simulink model "01_zvzvsspd"  (R2025a)
settings: Solver=FixedStepDiscrete  StartTime=0.0  StopTime=10  FixedStep=Ts  RelTol=1e-3
model workspace (MATLAB code in the model file):
  | N = 31;
  | n = 0:N-1;
  | sigma = (N-1)/6;
  | g = exp(-0.5*((n-(N-1)/2)/sigma).^2);
  | h = g / sum(g);
undefined symbols (not defined in the file): DiscIntNeverNeededParam, Ts
settings Model: Creator=wattanakhonvipanna  LastModifiedBy=wattanakhonvipanna

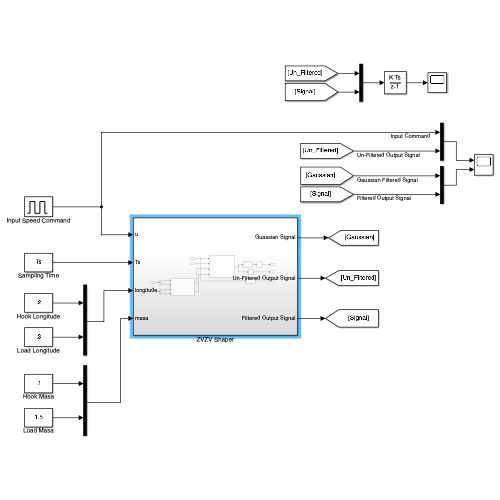
[thumbnail: Simulink's stored preview of the top-level diagram]
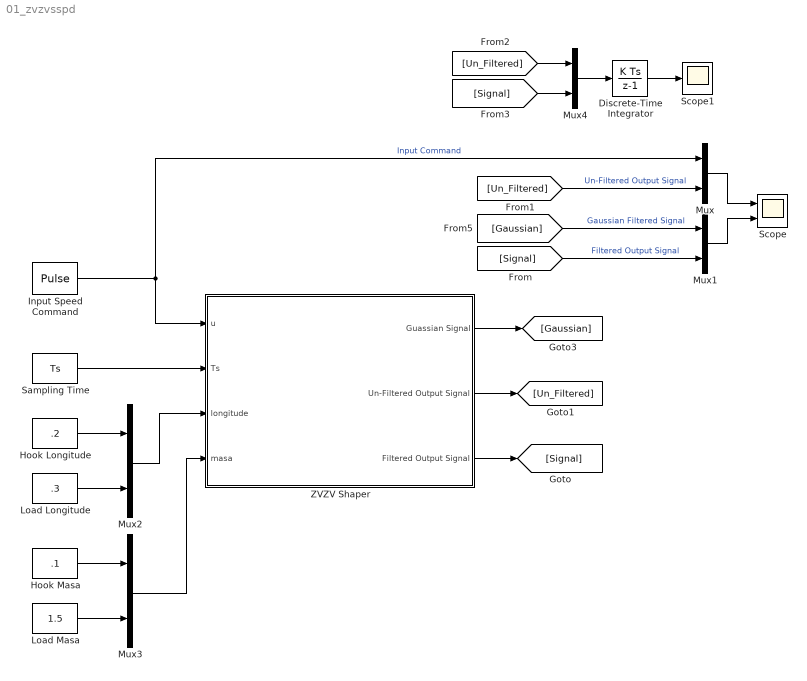
== system 01_zvzvsspd ==
  Discrete-Time Integrator : DiscreteIntegrator  SampleTime=-1  ICPrevOutput=DiscIntNeverNeededParam  ICPrevScaledInput=DiscIntNeverNeededParam
  Hook Longitude : Constant  Value=.2
  Hook Masa : Constant  Value=.1
  Input Speed Command : DiscretePulseGenerator  PulseType=Time based  Amplitude=0.2  Period=10  PulseWidth=50
  Load Longitude : Constant  Value=.3
  Load Masa : Constant  Value=1.5
  Mux{,1..4} (5 alike) : Mux  Inputs=2
  Sampling Time : Constant  Value=Ts
  Scope : Scope  NumInputPorts=2
      settings: ActiveDisplayYMinimum=-0.024999999999999998  ActiveDisplayYMaximum=0.22500000000000003  YLabel=speed (ms^-^1)
  Scope1 : Scope
      settings: ActiveDisplayYMinimum=-0.31249999999999656  ActiveDisplayYMaximum=2.8124999999999694  YLabel=position (m)  DataLoggingVariableName=ScopeData2
  ZVZV Shaper : Subsystem
  wires:
  Sampling Time/1 -> ZVZV Shaper/2(Ts)
  ZVZV Shaper/3(Filtered Output Signal) -> [Signal]
  ZVZV Shaper/2(Un-Filtered Output Signal) -> [Un_Filtered]
  [Un_Filtered] -> Mux/2  "Un-Filtered Output Signal"
  Mux/1 -> Scope/1
  Input Speed Command/1 -> ZVZV Shaper/1(u), Mux/1  "Input Command"
  Mux1/1 -> Scope/2
  [Gaussian] -> Mux1/1  "Gaussian Filtered Signal"
  [Signal] -> Mux1/2  "Filtered Output Signal"
  ZVZV Shaper/1(Guassian Signal) -> [Gaussian]
  Mux2/1 -> ZVZV Shaper/3(longitude)
  Hook Longitude/1 -> Mux2/1
  Load Longitude/1 -> Mux2/2
  Load Masa/1 -> Mux3/2
  Hook Masa/1 -> Mux3/1
  Mux3/1 -> ZVZV Shaper/4(masa)
  Mux4/1 -> Discrete-Time Integrator/1
  [Un_Filtered] -> Mux4/1
  [Signal] -> Mux4/2
  Discrete-Time Integrator/1 -> Scope1/1

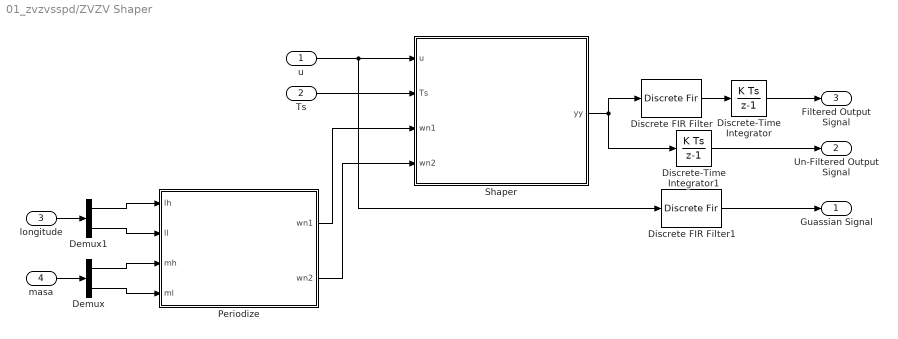
== system 01_zvzvsspd/ZVZV Shaper ==
  u : Inport
  Ts : Inport  Port=2
  longitude : Inport  Port=3
  masa : Inport  Port=4
  Demux : Demux  Outputs=2
  Demux1 : Demux  Outputs=2
  Discrete FIR Filter : DiscreteFir  Coefficients=h
  Discrete FIR Filter1 : DiscreteFir  Coefficients=h
  Discrete-Time Integrator : DiscreteIntegrator  SampleTime=Ts  ICPrevOutput=DiscIntNeverNeededParam  ICPrevScaledInput=DiscIntNeverNeededParam
  Discrete-Time Integrator1 : DiscreteIntegrator  SampleTime=Ts  ICPrevOutput=DiscIntNeverNeededParam  ICPrevScaledInput=DiscIntNeverNeededParam
  Periodize : MATLAB Function  TreatAsAtomicUnit=on
  Shaper : MATLAB Function  TreatAsAtomicUnit=on
  Guassian Signal : Outport
  Un-Filtered Output Signal : Outport  Port=2
  Filtered Output Signal : Outport  Port=3
  wires:
  u/1 -> Discrete FIR Filter1/1, Shaper/1(u)
  Ts/1 -> Shaper/2(Ts)
  Discrete-Time Integrator/1 -> Filtered Output Signal/1
  Shaper/1(yy) -> Discrete-Time Integrator1/1, Discrete FIR Filter/1
  Discrete FIR Filter/1 -> Discrete-Time Integrator/1
  Discrete-Time Integrator1/1 -> Un-Filtered Output Signal/1
  Discrete FIR Filter1/1 -> Guassian Signal/1
  masa/1 -> Demux/1
  longitude/1 -> Demux1/1
  Demux1/1 -> Periodize/1(lh)
  Demux1/2 -> Periodize/2(ll)
  Demux/1 -> Periodize/3(mh)
  Demux/2 -> Periodize/4(ml)
  Periodize/1(wn1) -> Shaper/3(wn1)
  Periodize/2(wn2) -> Shaper/4(wn2)

== matlab function 01_zvzvsspd/ZVZV Shaper/Periodize ==
  data: lh input; ll input; mh input; wn1 output; wn2 output; ml input
function [wn1, wn2]= ModePeriodize(lh, ll, mh, ml)

g = 9.81;

a = mh * lh * ll;
b = (mh * g * ll) + (ml * g * ll) + (mh * g * lh) + (ml * g * lh);
c = (mh * g * g) + (ml * g * g);

wn1 = sqrt((b - sqrt(b * b - 4 * a * c))/ (2 * a));
wn2 = sqrt((b + sqrt(b * b - 4 * a * c))/ (2 * a));

== matlab function 01_zvzvsspd/ZVZV Shaper/Shaper ==
  data: u input; yy output; Ts input; wn1 input; wn2 input
function yy = ZVZVshaper(u, Ts, wn1, wn2)

persistent armed k last_u A_tot d2 d3 d4
if isempty(armed)
    armed  = false;
    k      = double(0);
    last_u = 0.0;
    A_tot  = 0.0;
    d2     = double(0);
    d3     = double(0);
    d4     = double(0);
end

yy = 0.0;                
tol = 1e-12;

du = u - last_u;
last_u = u;

if ~armed && (abs(du) > tol)
    A_tot = du;
    k     = double(0);
    T1    = 2*pi / max(wn1, 1e-9);
    T2    = 2*pi / max(wn2, 1e-9);
    d2    = double( round( (0.5*T2) / max(Ts,1e-12) ) ); 
    d3    = double( round( (0.5*T1) / max(Ts,1e-12) ) );
    d4    = double( round( (0.5*(T1 + T2)) / max(Ts,1e-12) ) );
    armed = true;
end


if armed
    if k == double(0)
        yy = (0.25*A_tot)  / max(Ts,1e-12);
    elseif k == d2
        yy = (0.25*A_tot)  / max(Ts,1e-12);
    elseif k == d3
        yy = (0.25*A_tot)  / max(Ts,1e-12);
    elseif k == d4
        yy = (0.25*A_tot)  / max(Ts,1e-12);
    end

    k = k + double(1);
    if k > d4 + double(1)
        armed = false;
    end
end
